simulink model "sensitivity_th"  (R2018b)
settings: Solver=ode8  StartTime=0.0  StopTime=end_time  FixedStep=1  RelTol=1e-3
values from neighbouring files (symbols this model uses):
  botDotMean = mean(botDot(:,:,sampleSize:end),3)    [sensitivity.m]
  sideDotMean = mean(sideDot(:,:,sampleSize:end),3)    [sensitivity.m]
  slntDotMean = mean(slntDot(:,:,sampleSize:end),3)    [sensitivity.m]
undefined symbols (not defined in the file or in its folder): getVal
libraries: find6DOF_cl x1
settings Model: Creator=mae-ncsucore  LastModifiedBy=mae-ncsucore

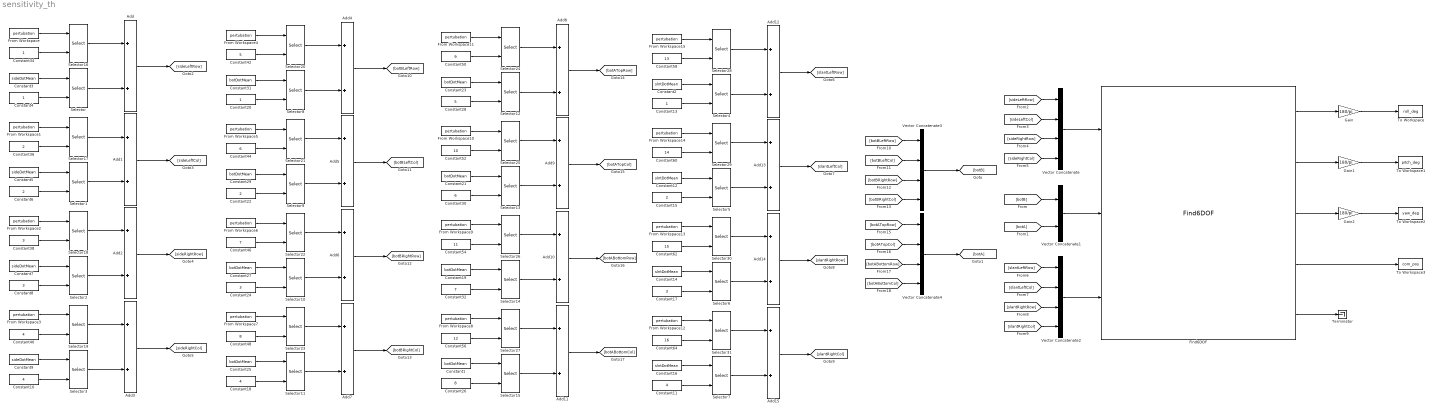
== system sensitivity_th ==
  Add{,1..15} (16 alike) : Sum
  Constant{1,19,21,23,25,27,29,31} (8 alike) : Constant  Value=botDotMean
  Constant{10..11,18,40} (4 alike) : Constant  Value=4
  Constant{2,12,14,16} (4 alike) : Constant  Value=slntDotMean
  Constant{4,13,20,34} (4 alike) : Constant
  Constant{6,15,22,36} (4 alike) : Constant  Value=2
  Constant{8,17,24,38} (4 alike) : Constant  Value=3
  Constant26 : Constant  Value=8
  Constant28 : Constant  Value=5
  Constant{3,5,7,9} (4 alike) : Constant  Value=sideDotMean
  Constant30 : Constant  Value=6
  Constant32 : Constant  Value=7
  Constant42 : Constant  Value=5
  Constant44 : Constant  Value=6
  Constant46 : Constant  Value=7
  Constant48 : Constant  Value=8
  Constant50 : Constant  Value=9
  Constant52 : Constant  Value=10
  Constant54 : Constant  Value=11
  Constant56 : Constant  Value=12
  Constant58 : Constant  Value=13
  Constant60 : Constant  Value=14
  Constant62 : Constant  Value=15
  Constant64 : Constant  Value=16
  Find6DOF : find6DOF_cl/Find6DOF  imageDims_px=getVal('sideImageSize_px')  initialCoMPositionVec_cm=getVal('initCoMPosVec_cm')  cameraFOVAngles_deg=getVal('cameraFOV_deg')  sideEulerAngles=getVal('sideCamEulAng_deg')  sideCamPositionVec_cm=getVal('sideCamPosVec_cm')  botEulerAngles=getVal('botCamEulAng_deg')  botCamPositionVec_cm=getVal('botCamPosVec_cm')  slantEulerAngles=getVal('slntCamEulAng_deg')  slantCamPositionVec_cm=getVal('slntCamPosVec_cm')  sideSeparation_cm=getVal('sideDotSepDist_cm')  sidePositionVecBF_cm=getVal('sideDotPosVec_cm')  bottomASeparation_cm=getVal('botADotSepDist_cm')  botAPositionVecBF_cm=getVal('botADotPosVec_cm')  bottomBSeparation_cm=getVal('botBDotSepDist_cm')  botBPositionVecBG_cm=getVal('botBDotPosVec_cm')
  From Workspace{,1..15} (16 alike) : FromWorkspace  VariableName=pertubation  SampleTime=0
  Gain : Gain  Gain=180/pi
  Gain1 : Gain  Gain=180/pi
  Gain2 : Gain  Gain=180/pi
  Selector{,1..7} (8 alike) : Selector  InputPortWidth=4  IndexOptions=Starting index (port)  Indices=[1 3]  OutputSizes=1
  Selector{8..15} (8 alike) : Selector  InputPortWidth=8  IndexOptions=Starting index (port)  Indices=[1 3]  OutputSizes=1
  Selector{16..31} (16 alike) : Selector  InputPortWidth=16  IndexOptions=Starting index (port)  Indices=[1 3]  OutputSizes=1
  Terminator : Terminator
  To Workspace : ToWorkspace  VariableName=roll_deg  SaveFormat=Timeseries  SampleTime=-1
  To Workspace1 : ToWorkspace  VariableName=pitch_deg  SaveFormat=Timeseries  SampleTime=-1
  To Workspace2 : ToWorkspace  VariableName=yaw_deg  SaveFormat=Timeseries  SampleTime=-1
  To Workspace3 : ToWorkspace  VariableName=com_pos  SaveFormat=Timeseries  SampleTime=-1
  Vector Concatenate{,2..4} (4 alike) : Concatenate  NumInputs=4
  Vector Concatenate1 : Concatenate
  wires:
  Find6DOF/3 -> Gain2/1
  Find6DOF/2 -> Gain1/1
  Find6DOF/1 -> Gain/1
  Gain/1 -> To Workspace/1
  Gain1/1 -> To Workspace1/1
  Gain2/1 -> To Workspace2/1
  Find6DOF/4 -> To Workspace3/1
  Vector Concatenate/1 -> Find6DOF/1
  Vector Concatenate2/1 -> Find6DOF/3
  Vector Concatenate1/1 -> Find6DOF/2
  [botB] -> Vector Concatenate1/1
  [botA] -> Vector Concatenate1/2
  [slantRightRow] -> Vector Concatenate2/3
  [slantRightCol] -> Vector Concatenate2/4
  [slantLeftCol] -> Vector Concatenate2/2
  [slantLeftRow] -> Vector Concatenate2/1
  [sideRightCol] -> Vector Concatenate/4
  [sideRightRow] -> Vector Concatenate/3
  [sideLeftCol] -> Vector Concatenate/2
  [sideLeftRow] -> Vector Concatenate/1
  Vector Concatenate3/1 -> [botB]
  Vector Concatenate4/1 -> [botA]
  [botBLeftRow] -> Vector Concatenate3/1
  [botBLeftCol] -> Vector Concatenate3/2
  [botBRightRow] -> Vector Concatenate3/3
  [botBRightCol] -> Vector Concatenate3/4
  [botATopRow] -> Vector Concatenate4/1
  [botATopCol] -> Vector Concatenate4/2
  [botABottomRow] -> Vector Concatenate4/3
  [botABottomCol] -> Vector Concatenate4/4
  Constant3/1 -> Selector/1
  Constant4/1 -> Selector/2
  Constant6/1 -> Selector1/2
  Constant5/1 -> Selector1/1
  Constant7/1 -> Selector2/1
  Constant8/1 -> Selector2/2
  Constant10/1 -> Selector3/2
  Constant9/1 -> Selector3/1
  Constant15/1 -> Selector5/2
  Constant14/1 -> Selector6/1
  Constant17/1 -> Selector6/2
  Constant13/1 -> Selector4/2
  Constant16/1 -> Selector7/1
  Constant11/1 -> Selector7/2
  Constant12/1 -> Selector5/1
  Constant2/1 -> Selector4/1
  Constant22/1 -> Selector9/2
  Constant27/1 -> Selector10/1
  Constant24/1 -> Selector10/2
  Constant20/1 -> Selector8/2
  Constant25/1 -> Selector11/1
  Constant18/1 -> Selector11/2
  Constant29/1 -> Selector9/1
  Constant31/1 -> Selector8/1
  Constant30/1 -> Selector13/2
  Constant19/1 -> Selector14/1
  Constant32/1 -> Selector14/2
  Constant28/1 -> Selector12/2
  Constant1/1 -> Selector15/1
  Constant26/1 -> Selector15/2
  Constant21/1 -> Selector13/1
  Constant23/1 -> Selector12/1
  From Workspace/1 -> Selector16/1
  Add/1 -> [sideLeftRow]
  Constant34/1 -> Selector16/2
  Selector/1 -> Add/2
  Selector16/1 -> Add/1
  Selector17/1 -> Add1/1
  Constant36/1 -> Selector17/2
  From Workspace1/1 -> Selector17/1
  Add1/1 -> [sideLeftCol]
  Selector1/1 -> Add1/2
  Selector18/1 -> Add2/1
  From Workspace2/1 -> Selector18/1
  Constant38/1 -> Selector18/2
  Add2/1 -> [sideRightRow]
  Selector2/1 -> Add2/2
  Constant40/1 -> Selector19/2
  From Workspace3/1 -> Selector19/1
  Selector19/1 -> Add3/1
  Selector3/1 -> Add3/2
  Add3/1 -> [sideRightCol]
  Selector20/1 -> Add4/1
  From Workspace4/1 -> Selector20/1
  Constant42/1 -> Selector20/2
  Add4/1 -> [botBLeftRow]
  Selector8/1 -> Add4/2
  From Workspace5/1 -> Selector21/1
  Constant44/1 -> Selector21/2
  Selector21/1 -> Add5/1
  Add5/1 -> [botBLeftCol]
  Selector9/1 -> Add5/2
  From Workspace6/1 -> Selector22/1
  Constant46/1 -> Selector22/2
  Selector22/1 -> Add6/1
  Add6/1 -> [botBRightRow]
  Selector10/1 -> Add6/2
  From Workspace7/1 -> Selector23/1
  Constant48/1 -> Selector23/2
  Selector23/1 -> Add7/1
  Add7/1 -> [botBRightCol]
  Selector11/1 -> Add7/2
  From Workspace11/1 -> Selector24/1
  Constant50/1 -> Selector24/2
  Selector24/1 -> Add8/1
  Add8/1 -> [botATopRow]
  Selector12/1 -> Add8/2
  From Workspace10/1 -> Selector25/1
  Constant52/1 -> Selector25/2
  Selector25/1 -> Add9/1
  Selector13/1 -> Add9/2
  Add9/1 -> [botATopCol]
  From Workspace9/1 -> Selector26/1
  Constant54/1 -> Selector26/2
  Selector26/1 -> Add10/1
  Add10/1 -> [botABottomRow]
  Selector14/1 -> Add10/2
  From Workspace8/1 -> Selector27/1
  Constant56/1 -> Selector27/2
  Selector27/1 -> Add11/1
  Add11/1 -> [botABottomCol]
  Selector15/1 -> Add11/2
  From Workspace15/1 -> Selector28/1
  Constant58/1 -> Selector28/2
  Selector28/1 -> Add12/1
  Selector4/1 -> Add12/2
  Add12/1 -> [slantLeftRow]
  From Workspace14/1 -> Selector29/1
  Constant60/1 -> Selector29/2
  Selector29/1 -> Add13/1
  Add13/1 -> [slantLeftCol]
  Selector5/1 -> Add13/2
  From Workspace13/1 -> Selector30/1
  Constant62/1 -> Selector30/2
  Selector30/1 -> Add14/1
  Add14/1 -> [slantRightRow]
  Selector6/1 -> Add14/2
  From Workspace12/1 -> Selector31/1
  Constant64/1 -> Selector31/2
  Selector31/1 -> Add15/1
  Add15/1 -> [slantRightCol]
  Selector7/1 -> Add15/2
  Find6DOF/5 -> Terminator/1
